simulink model "TaperedTLMExample"  (R2015a)
settings: Solver=ode23t  StartTime=0.0  StopTime=2  RelTol=1e-6
libraries: usask_tlm_lib x1
settings Model: Creator=Jeremy  LastModifiedBy=tkw954
settings DataIOCC: LimitDataPoints=off

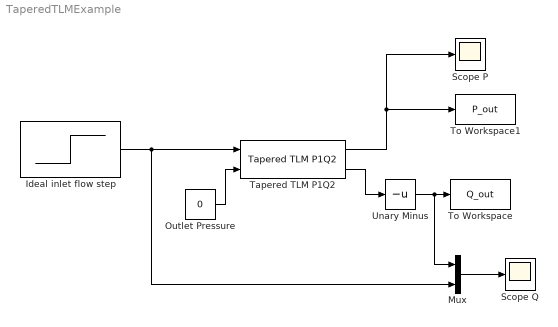
== system TaperedTLMExample ==
  Ideal inlet flow step : Step  After=2.5e-4  SampleTime=0
  Mux : Mux  Inputs=2
  Outlet Pressure : Constant  Value=0
  Scope P : Scope
      settings: TimeRange=2  YMin=0  YMax=2
  Scope Q : Scope
      settings: TimeRange=0.0110489915596052  YMin=-2e-07  YMax=2e-07
  Tapered TLM P1Q2 : usask_tlm_lib/Tapered TLM P1Q2  D_1=40e-3  D_2=42e-3  L=10  K=1.5e9  nu=100e-6  rho=890
  To Workspace : ToWorkspace  VariableName=Q_out  SampleTime=-1
  To Workspace1 : ToWorkspace  VariableName=P_out  SampleTime=-1
  Unary Minus : UnaryMinus
  wires:
  Ideal inlet flow step/1 -> Mux/2, Tapered TLM P1Q2/1
  Outlet Pressure/1 -> Tapered TLM P1Q2/2
  Tapered TLM P1Q2/1 -> To Workspace1/1, Scope P/1
  Unary Minus/1 -> Mux/1, To Workspace/1
  Mux/1 -> Scope Q/1
  Tapered TLM P1Q2/2 -> Unary Minus/1
